simulink model "question4"  (R2023b)
settings: Solver=VariableStepAuto  StartTime=0.0  StopTime=10  RelTol=1e-3
values from neighbouring files (symbols this model uses):
  A = [-8.8487+(a-b)/5,-0.0399,-5.55+(c+d)/10,3.5846 ... (first row only)    [main_func.m]    (also in question3.m = [-8.8487+(a-b)/5, -0.0399, -5.55+(c+d)/10, 3.5846)
  B = [0.0564+b/(10+c),0.0319 ... (first row only)    [main_func.m]    (also in question3.m = [0.0564+b/(10+c), 0.0319)
  C = [-3.2988,-2.1932+(10*c+d)/(100+5*a),0.037,-0.0109 ... (first row only)    [main_func.m]    (also in question3.m = [-3.2988, -2.1932+(10*c+d)/(100+5*a), 0.037, -0.0109)
  F = inv(B_star)    [main_func.m]
  K_4 = inv(B_star) * C_star2    [main_func.m]
  x0 = [0.5;-0.1;0.3;-0.8]    [main_func.m]    (also in question3.m = [0.5; -0.1; 0.3; -0.8])
settings Model: Creator=Fan Xiuqi  LastModifiedBy=Fan Xiuqi

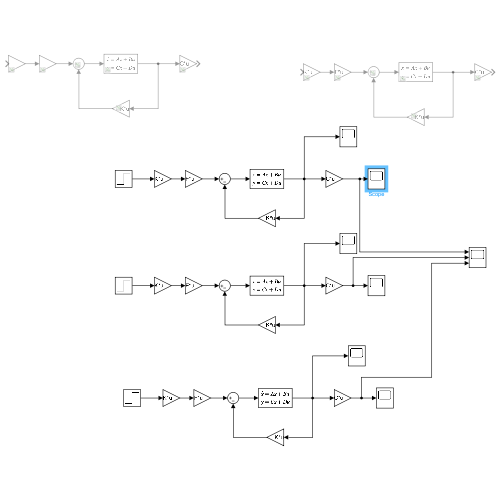
[thumbnail: Simulink's stored preview of the top-level diagram]
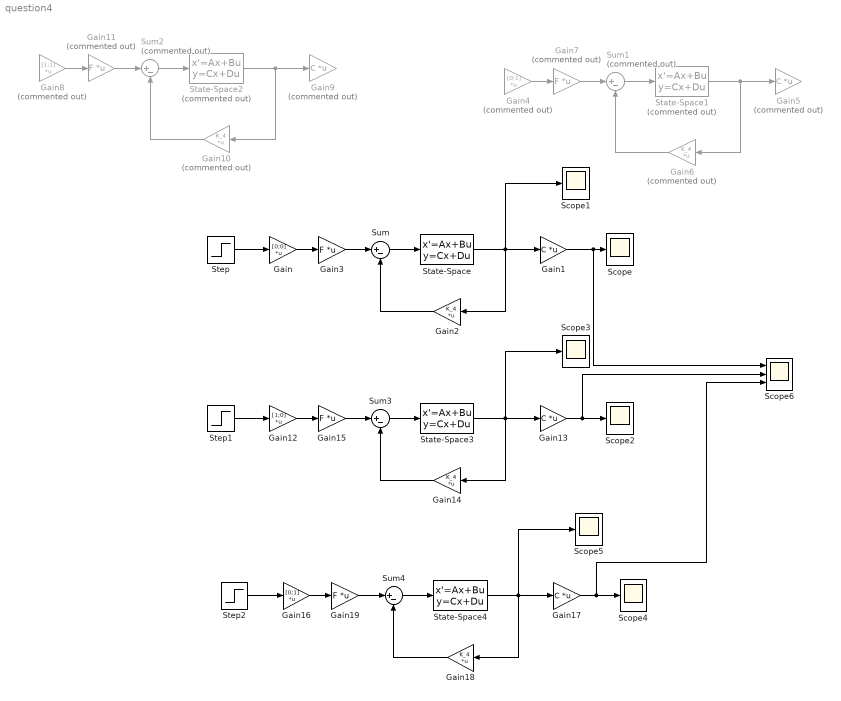
== system question4 ==
  Gain : Gain  Gain=[0;0]  Multiplication=Matrix(K*u)
  Gain1 : Gain  Gain=C  Multiplication=Matrix(K*u)
  Gain10 : Gain  Commented=on  Gain=K_4  Multiplication=Matrix(K*u)
  Gain11 : Gain  Commented=on  Gain=F  Multiplication=Matrix(K*u)
  Gain12 : Gain  Gain=[1;0]  Multiplication=Matrix(K*u)
  Gain13 : Gain  Gain=C  Multiplication=Matrix(K*u)
  Gain14 : Gain  Gain=K_4  Multiplication=Matrix(K*u)
  Gain15 : Gain  Gain=F  Multiplication=Matrix(K*u)
  Gain16 : Gain  Gain=[0;1]  Multiplication=Matrix(K*u)
  Gain17 : Gain  Gain=C  Multiplication=Matrix(K*u)
  Gain18 : Gain  Gain=K_4  Multiplication=Matrix(K*u)
  Gain19 : Gain  Gain=F  Multiplication=Matrix(K*u)
  Gain2 : Gain  Gain=K_4  Multiplication=Matrix(K*u)
  Gain3 : Gain  Gain=F  Multiplication=Matrix(K*u)
  Gain4 : Gain  Commented=on  Gain=[0;1]  Multiplication=Matrix(K*u)
  Gain5 : Gain  Commented=on  Gain=C  Multiplication=Matrix(K*u)
  Gain6 : Gain  Commented=on  Gain=K_4  Multiplication=Matrix(K*u)
  Gain7 : Gain  Commented=on  Gain=F  Multiplication=Matrix(K*u)
  Gain8 : Gain  Commented=on  Gain=[1;1]  Multiplication=Matrix(K*u)
  Gain9 : Gain  Commented=on  Gain=C  Multiplication=Matrix(K*u)
  Scope{,1..5} (6 alike) : Scope
  Scope6 : Scope  NumInputPorts=3
  State-Space : StateSpace  A=A  B=B  C=eye(4)  D=zeros(4,2)  InitialCondition=x0
  State-Space1 : StateSpace  Commented=on  A=A  B=B  C=eye(4)  D=zeros(4,2)  InitialCondition=0
  State-Space2 : StateSpace  Commented=on  A=A  B=B  C=eye(4)  D=zeros(4,2)  InitialCondition=0
  State-Space3 : StateSpace  A=A  B=B  C=eye(4)  D=zeros(4,2)  InitialCondition=0
  State-Space4 : StateSpace  A=A  B=B  C=eye(4)  D=zeros(4,2)  InitialCondition=0
  Step : Step  SampleTime=0
  Step1 : Step  SampleTime=0
  Step2 : Step  SampleTime=0
  Sum : Sum  Inputs=|+-
  Sum1 : Sum  Commented=on  Inputs=|+-
  Sum2 : Sum  Commented=on  Inputs=|+-
  Sum3 : Sum  Inputs=|+-
  Sum4 : Sum  Inputs=|+-
  wires:
  Step/1 -> Gain/1
  Gain/1 -> Gain3/1
  Sum/1 -> State-Space/1
  Gain1/1 -> Scope6/1, Scope/1
  State-Space/1 -> Gain2/1, Scope1/1, Gain1/1
  Gain2/1 -> Sum/2
  Gain3/1 -> Sum/1
  Gain7/1 -> Sum1/1
  Sum1/1 -> State-Space1/1
  Gain6/1 -> Sum1/2
  State-Space1/1 -> Gain6/1, Gain5/1
  Gain4/1 -> Gain7/1
  Gain11/1 -> Sum2/1
  Sum2/1 -> State-Space2/1
  State-Space2/1 -> Gain10/1, Gain9/1
  Gain10/1 -> Sum2/2
  Gain8/1 -> Gain11/1
  Step1/1 -> Gain12/1
  State-Space3/1 -> Gain14/1, Scope3/1, Gain13/1
  Gain12/1 -> Gain15/1
  Gain14/1 -> Sum3/2
  Gain15/1 -> Sum3/1
  Gain13/1 -> Scope6/2, Scope2/1
  Sum3/1 -> State-Space3/1
  Step2/1 -> Gain16/1
  State-Space4/1 -> Gain18/1, Scope5/1, Gain17/1
  Gain16/1 -> Gain19/1
  Gain18/1 -> Sum4/2
  Gain19/1 -> Sum4/1
  Gain17/1 -> Scope6/3, Scope4/1
  Sum4/1 -> State-Space4/1
